simulink model "VectorSensor"  (R2019b)
settings: configuration reference "cset" (kept outside this file)
PostLoadFcn:
  | disp(['Executing PostLoadFcn in ' get_param(gcs,'Name')])
  | 
  | % Resize bus objects
  | hws = get_param(gcs, 'modelworkspace');
  | [SonarWorkbenchElementObj,SonarWorkbenchArrayObj,SonarWorkbenchBeamObj] = SetAcousticSensorDesignDimensions(hws.getVariable('Ne'),hws.getVariable('Ntype'),SonarWorkbenchElementObj,SonarWorkbenchArrayObj,SonarWorkbenchBeamObj);
  | clear hws
model workspace (MAT data in the model file):
  Ne = 4
  Ntype = 2
settings Model: Creator=tom  LastModifiedBy=tom
settings ConfigSetRef: SourceName=cset  SourceLocation=Base Workspace

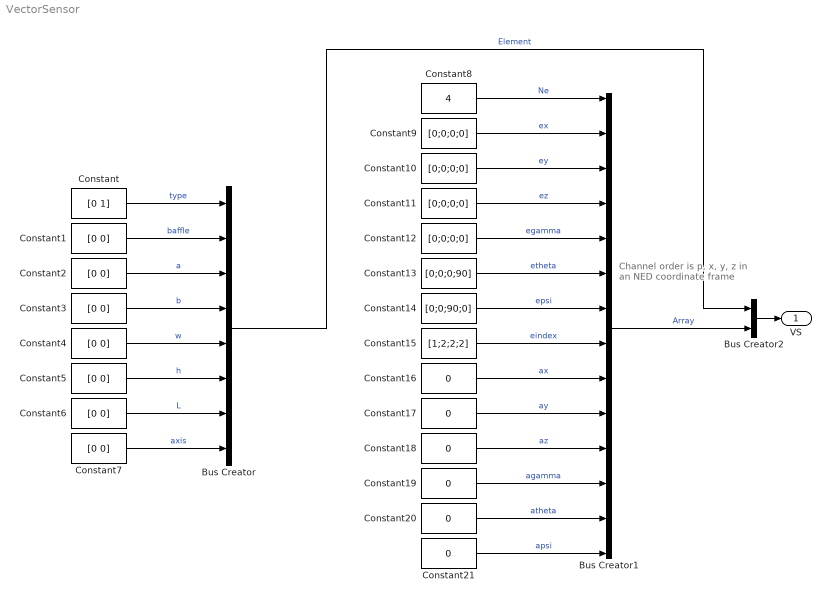
== system VectorSensor ==
  note: Channel order is p, x, y, z in an NED coordinate frame
  Bus Creator : BusCreator  Inputs=8  OutDataTypeStr=Bus: SonarWorkbenchElementObj
  Bus Creator1 : BusCreator  Inputs=14  OutDataTypeStr=Bus: SonarWorkbenchArrayObj
  Bus Creator2 : BusCreator  Inputs=2  OutDataTypeStr=Bus: SonarWorkbenchAcousticSensorObj
  Constant : Constant  Value=[0 1]  VectorParams1D=off  OutDataTypeStr=int32
  Constant{1..7} (7 alike) : Constant  Value=[0 0]  VectorParams1D=off  OutDataTypeStr=double
  Constant{9..12} (4 alike) : Constant  Value=[0;0;0;0]  VectorParams1D=off  OutDataTypeStr=double
  Constant13 : Constant  Value=[0;0;0;90]  VectorParams1D=off  OutDataTypeStr=double
  Constant14 : Constant  Value=[0;0;90;0]  VectorParams1D=off  OutDataTypeStr=double
  Constant15 : Constant  Value=[1;2;2;2]  VectorParams1D=off  OutDataTypeStr=double
  Constant{16..21} (6 alike) : Constant  Value=0  VectorParams1D=off  OutDataTypeStr=double
  Constant8 : Constant  Value=4  VectorParams1D=off  OutDataTypeStr=int32
  VS : Outport  OutDataTypeStr=Bus: SonarWorkbenchAcousticSensorObj
  wires:
  Constant/1 -> Bus Creator/1  "type"
  Constant1/1 -> Bus Creator/2  "baffle"
  Constant2/1 -> Bus Creator/3  "a"
  Constant3/1 -> Bus Creator/4  "b"
  Constant4/1 -> Bus Creator/5  "w"
  Constant5/1 -> Bus Creator/6  "h"
  Constant6/1 -> Bus Creator/7  "L"
  Constant7/1 -> Bus Creator/8  "axis"
  Bus Creator/1 -> Bus Creator2/1  "Element"
  Constant8/1 -> Bus Creator1/1  "Ne"
  Constant9/1 -> Bus Creator1/2  "ex"
  Constant10/1 -> Bus Creator1/3  "ey"
  Constant11/1 -> Bus Creator1/4  "ez"
  Constant12/1 -> Bus Creator1/5  "egamma"
  Constant13/1 -> Bus Creator1/6  "etheta"
  Constant14/1 -> Bus Creator1/7  "epsi"
  Constant15/1 -> Bus Creator1/8  "eindex"
  Constant16/1 -> Bus Creator1/9  "ax"
  Constant17/1 -> Bus Creator1/10  "ay"
  Constant18/1 -> Bus Creator1/11  "az"
  Constant19/1 -> Bus Creator1/12  "agamma"
  Constant20/1 -> Bus Creator1/13  "atheta"
  Constant21/1 -> Bus Creator1/14  "apsi"
  Bus Creator1/1 -> Bus Creator2/2  "Array"
  Bus Creator2/1 -> VS/1
